simulink model "cpp_m1hp_demo"  (R2022b)
settings: Solver=FixedStepDiscrete  StartTime=0.0  StopTime=6  FixedStep=FEM_Ts  MaxStep=FEM_Ts  RelTol=1e-2
InitFcn:
  | %
  | % Initialization callback function
  | %
  | 
  | try
  |    fprintf('\nGMT IMS version (%s)!\n',simulink_fname );
  | 
  |    % Get Simulink model directory
  |    [filepath,name,ext] = fileparts(which(bdroot));
  | 
  |    if ~strcmp(filepath,pwd)
  |       fprintf('\nChanging current directory to \n %s \n',filepath);
  |       cd(filepath);
  |    end
  | 
  |    %
  |  if(osim.bpless_wl)
  |     fprintf('Generating bumpless wind load time series\n');
  |  end
  | catch
  |    warning('Running the InitFcn from puSimulate script');
  | end
values from neighbouring files (symbols this model uses):
  a_max = 250e-6    (= 0.00025)    [load_im_with_m1act_damp.m]    (also in load_m1hp_cpp_demo.m)
  b = B(:,in)*m1sys{seg}.Kbal    [evalM1ofl_act_damp.m]
  c = [Upsilon*C(out0,:);     C(out1a,:)-C(out1b,:);     C(out2,:)]    [evalM1ofl_act_damp.m]
  delta_sim = 1e-3    (= 0.001)    [load_im_with_m1act_damp.m]    (also in load_m1hp_cpp_demo.m)
  drv_delay = ceil(mount.delay/FEM_Ts)    [load_im_with_m1act_damp.m]    (also in load_m1hp_cpp_demo.m)
  FEM_Ts = 1/1e3    (= 0.001)    [load_im_with_m1act_damp.m]    (also in load_m1hp_cpp_demo.m)
  Hdrive_d = c2d(o.Hdrive(1,1), FEM_Ts, 'tustin')    [load_im_with_m1act_damp.m]    (also in load_m1hp_cpp_demo.m)
  m1sys = ovr_ofl_crtl(m1sys,seg)    [evalM1ofl_act_damp.m]    (also in load_im_with_m1act_damp.m = ovr_ofl_crtl(m1sys))
  o = fun_confBase(oTest)    [load_im_with_m1act_damp.m]    (also in load_m1hp_cpp_demo.m)
  PG = zeros(length(om2),6)    [load_im_with_m1act_damp.m]    (also in load_m1hp_cpp_demo.m)
  phiB = inputs2ModalF(mode_ind_vec,indDesInputs)    [load_im_with_m1act_damp.m]    (also in load_m1hp_cpp_demo.m)
  phiC = modalDisp2Outputs(indDesOutputs,mode_ind_vec)    [load_im_with_m1act_damp.m]    (also in load_m1hp_cpp_demo.m)
  Psi_ss = gainMatrix(indDesOutputs,indDesInputs) - K_ss    [load_im_with_m1act_damp.m]    (also in load_m1hp_cpp_demo.m)
  t_gd = 0*0.5    (= 0)    [load_im_with_m1act_damp.m]    (also in load_m1hp_cpp_demo.m)
  t_gd_v = 0*t_gd    (= 0)    [load_im_with_m1act_damp.m]    (also in load_m1hp_cpp_demo.m)
  Tcmd = 12    [load_im_with_m1act_damp.m]    (also in load_m1hp_cpp_demo.m)
  v0 = 0    [load_im_with_m1act_damp.m]    (also in load_m1hp_cpp_demo.m)
  v_max = 50e-6    (= 5e-05)    [load_im_with_m1act_damp.m]    (also in load_m1hp_cpp_demo.m)
  x0 = 0    [load_im_with_m1act_damp.m]    (also in load_m1hp_cpp_demo.m)
  x0_f = xf(end,:)    [load_im_with_m1act_damp.m]    (also in load_m1hp_cpp_demo.m)
undefined symbols (not defined in the file or in its folder): a, A_f, az, az_ff_en, B_f, C_f, D_f, DiscIntNeverNeededParam, el, gir, magnitude, mount, osim
libraries: simulink x8, ims_block_library x7, simulink_extras x2
(part 2 of 3)

== system cpp_m1hp_demo/M1 CPP/cmd_pre_proc/CPP with multi-axis coordination1 ==
  k : Inport
  k_acd : Inport  Port=2
  Demux1 : Demux  Outputs=3
  Dk_merge : Merge  Inputs=4  InitialOutput=0
  If Action Subsystem : Subsystem  TreatAsAtomicUnit=on
  If Action Subsystem1 : Subsystem  TreatAsAtomicUnit=on
  If Action Subsystem6 : Subsystem  TreatAsAtomicUnit=on
  If Action Subsystem__1 : Subsystem  TreatAsAtomicUnit=on
  If2 : If  NumInputs=2  IfExpression=(u1 == 0) | (u1 <= u2(1))  ElseIfExpressions=((u1 > u2(1)) & (u1 <= u2(2))), ((u1 > u2(2)) & (u1 <= u2(3))), (u1 > u2(3))  ShowElse=off
  Dk : Outport
  wires:
  k_acd/1 -> If2/2, Demux1/1
  k/1 -> If2/1
  Demux1/3 -> If Action Subsystem6/1(t_acd)
  If Action Subsystem__1/1(Dk) -> Dk_merge/3
  Demux1/1 -> If Action Subsystem1/1(t_a)
  If2/1 -> If Action Subsystem/Action
  If Action Subsystem/1(Dk) -> Dk_merge/1
  Demux1/2 -> If Action Subsystem__1/1(t_ac)
  If Action Subsystem1/1(Dk) -> Dk_merge/2
  If Action Subsystem6/1(Dk) -> Dk_merge/4
  Dk_merge/1 -> Dk/1
  If2/2 -> If Action Subsystem1/Action
  If2/3 -> If Action Subsystem__1/Action
  If2/4 -> If Action Subsystem6/Action

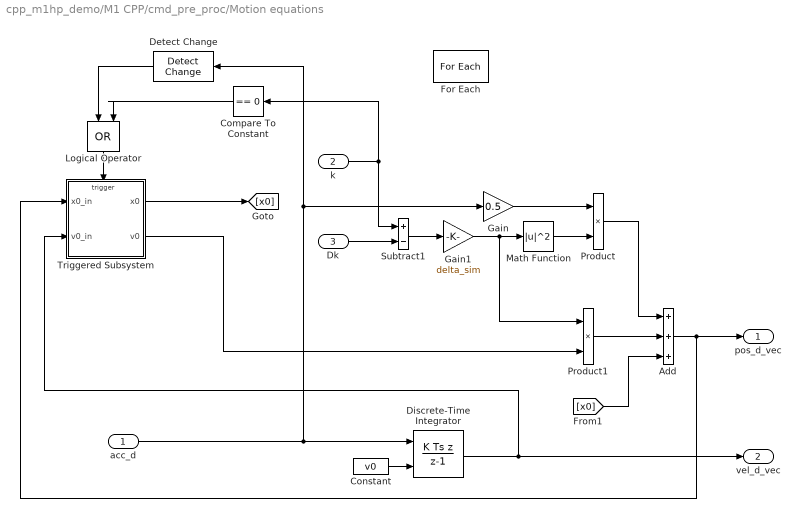
== system cpp_m1hp_demo/M1 CPP/cmd_pre_proc/Motion equations ==
  acc_d : Inport  Partition=on  PartitionDimension=1  PartitionWidth=1  PartitionOffset=0
  k : Inport  Port=2
  Dk : Inport  Port=3
  Add : Sum  Inputs=+++
  Compare To Constant : simulink/Logic and Bit Operations/Compare To Constant  relop===  const=0  OutDataTypeStr=boolean
  Constant : Constant  Value=v0
  Detect Change : simulink/Logic and Bit Operations/Detect Change  vinit=0  OutDataTypeStr=boolean
  Discrete-Time Integrator : DiscreteIntegrator  IntegratorMethod=Integration: Backward Euler  InitialConditionSource=external  InitialCondition=v0  SampleTime=-1  ICPrevOutput=DiscIntNeverNeededParam  ICPrevScaledInput=DiscIntNeverNeededParam
  For Each : ForEach  DisableCoverage=on
  Gain : Gain  Gain=0.5
  Gain1 : Gain  Gain=delta_sim  OutDataTypeStr=double
  Logical Operator : Logic  Operator=OR  IconShape=distinctive  AllPortsSameDT=off  OutDataTypeStr=boolean
  Math Function : Math  Operator=magnitude^2
  Product : Product
  Product1 : Product
  Subtract1 : Sum  Inputs=+-
  Triggered Subsystem : Subsystem  TreatAsAtomicUnit=on
  pos_d_vec : Outport  ConcatenationDimension=1
  vel_d_vec : Outport  Port=2  ConcatenationDimension=1
  wires:
  Detect Change/1 -> Logical Operator/1
  Add/1 -> pos_d_vec/1, Triggered Subsystem/1(x0_in)
  [x0] -> Add/3
  Gain/1 -> Product/1
  Constant/1 -> Discrete-Time Integrator/2
  Math Function/1 -> Product/2
  Triggered Subsystem/2(v0) -> Product1/2
  Product/1 -> Add/1
  acc_d/1 -> Discrete-Time Integrator/1, Gain/1, Detect Change/1
  Triggered Subsystem/1(x0) -> [x0]
  Discrete-Time Integrator/1 -> vel_d_vec/1, Triggered Subsystem/2(v0_in)
  Product1/1 -> Add/2
  k/1 -> Subtract1/1, Compare To Constant/1
  Gain1/1 -> Product1/1, Math Function/1
  Subtract1/1 -> Gain1/1
  Logical Operator/1 -> Triggered Subsystem/Trigger
  Compare To Constant/1 -> Logical Operator/2
  Dk/1 -> Subtract1/2

== system cpp_m1hp_demo/M1 CPP/cmd_pre_proc/Sample_generator ==
  Add : Sum
  Compare To Constant : simulink/Logic and Bit Operations/Compare To Constant  relop===  const=floor(Tcmd/delta_sim)  OutDataTypeStr=boolean
  Constant : Constant  OutDataTypeStr=uint32
  Resettable Delay : Delay  DelayLength=1  ExternalReset=Rising
      settings: InputPortMap=u0,r5
  Unit Delay : UnitDelay  SampleTime=-1  HasFrameUpgradeWarning=on
  k : Outport
  wires:
  Constant/1 -> Add/1
  Add/1 -> Resettable Delay/1, Unit Delay/1
  Resettable Delay/1 -> k/1, Add/2
  Compare To Constant/1 -> Resettable Delay/2
  Unit Delay/1 -> Compare To Constant/1

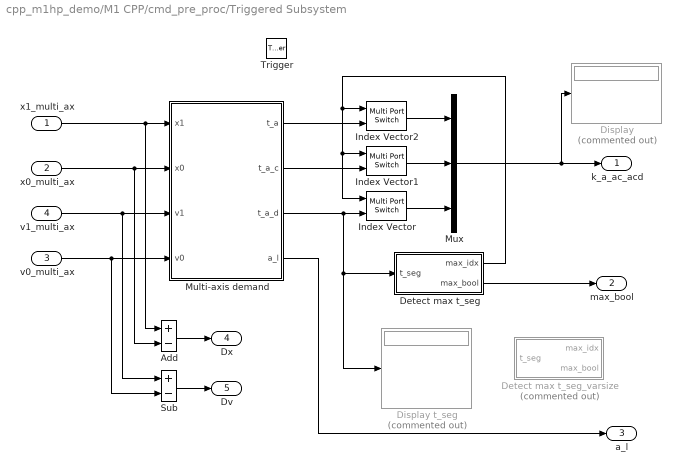
== system cpp_m1hp_demo/M1 CPP/cmd_pre_proc/Triggered Subsystem ==
  x1_multi_ax : Inport
  x0_multi_ax : Inport  Port=2  LatchByDelayingOutsideSignal=on
  v0_multi_ax : Inport  Port=3  LatchByDelayingOutsideSignal=on
  v1_multi_ax : Inport  Port=4
  Trigger : TriggerPort  VariantControl=Variant  InitialTriggerSignalState=zero
  Add : Sum  Inputs=+-
  Detect max t_seg : Subsystem
  Detect max t_seg_varsize : Subsystem  Commented=on
  Display : Display  Commented=on
  Display t_seg : Display  Commented=on
  Index Vector : MultiPortSwitch  Inputs=1  RndMeth=Simplest  SaturateOnIntegerOverflow=off
  Index Vector1 : MultiPortSwitch  Inputs=1  RndMeth=Simplest  SaturateOnIntegerOverflow=off
  Index Vector2 : MultiPortSwitch  Inputs=1  RndMeth=Simplest  SaturateOnIntegerOverflow=off
  Multi-axis demand : Subsystem  TreatAsAtomicUnit=on
  Mux : Mux  Inputs=3
  Sub : Sum  Inputs=+-
  k_a_ac_acd : Outport
  max_bool : Outport  Port=2
  a_l : Outport  Port=3
  Dx : Outport  Port=4
  Dv : Outport  Port=5
  wires:
  x1_multi_ax/1 -> Add/1, Multi-axis demand/1(x1)
  x0_multi_ax/1 -> Add/2, Multi-axis demand/2(x0)
  Detect max t_seg/1(max_idx) -> Index Vector1/1, Index Vector/1, Index Vector2/1
  v0_multi_ax/1 -> Sub/2, Multi-axis demand/4(v0)
  v1_multi_ax/1 -> Sub/1, Multi-axis demand/3(v1)
  Multi-axis demand/3(t_a_d) -> Index Vector/2, Display t_seg/1, Detect max t_seg/1(t_seg)
  Multi-axis demand/4(a_l) -> a_l/1
  Multi-axis demand/1(t_a) -> Index Vector2/2
  Multi-axis demand/2(t_a_c) -> Index Vector1/2
  Index Vector2/1 -> Mux/1
  Index Vector1/1 -> Mux/2
  Index Vector/1 -> Mux/3
  Mux/1 -> k_a_ac_acd/1, Display/1
  Add/1 -> Dx/1
  Sub/1 -> Dv/1
  Detect max t_seg/2(max_bool) -> max_bool/1

== system cpp_m1hp_demo/Mount_Drv_FDR2023_linear/DRV Friction/AZ DT Lugre Fr mode ==
  v : Inport
  Enable : EnablePort
  Constant : Constant  Value=iIsSig01Active
  Discrete-Time Integrator : DiscreteIntegrator  SampleTime=-1  ICPrevOutput=DiscIntNeverNeededParam  ICPrevScaledInput=DiscIntNeverNeededParam
  Sum : Sum  Inputs=+++
  g(v) : Subsystem
  sigma_0 : Gain  Gain=sigma0
  sigma_1 : Gain  Gain=sigma1
  sigma_v : Gain  Gain=sigmav
  v2z : Subsystem
  Tfr : Outport
  wires:
  Constant/1 -> g(v)/Enable, v2z/Enable
  v/1 -> sigma_v/1, v2z/1(v), g(v)/1(v)
  sigma_v/1 -> Sum/3
  sigma_1/1 -> Sum/1
  Sum/1 -> Tfr/1
  sigma_0/1 -> Sum/2
  g(v)/1(g) -> v2z/2(g(v))
  Discrete-Time Integrator/1 -> v2z/3(z), sigma_0/1
  v2z/1(dz) -> sigma_1/1, Discrete-Time Integrator/1

== system cpp_m1hp_demo/Mount_Drv_FDR2023_linear/DRV Friction/EL DT Lugre Fr model ==
  v : Inport
  Enable : EnablePort
  Constant : Constant  Value=iIsSig01Active
  Discrete-Time Integrator : DiscreteIntegrator  SampleTime=-1  ICPrevOutput=DiscIntNeverNeededParam  ICPrevScaledInput=DiscIntNeverNeededParam
  Sum : Sum  Inputs=+++
  g(v) : Subsystem
  sigma_0 : Gain  Gain=sigma0
  sigma_1 : Gain  Gain=sigma1
  sigma_v : Gain  Gain=sigmav
  v2z : Subsystem
  Tfr : Outport
  wires:
  Constant/1 -> g(v)/Enable, v2z/Enable
  sigma_0/1 -> Sum/2
  Discrete-Time Integrator/1 -> v2z/3(z), sigma_0/1
  g(v)/1(g) -> v2z/2(g(v))
  v/1 -> sigma_v/1, v2z/1(v), g(v)/1(v)
  Sum/1 -> Tfr/1
  sigma_1/1 -> Sum/1
  v2z/1(dz) -> sigma_1/1, Discrete-Time Integrator/1
  sigma_v/1 -> Sum/3

== system cpp_m1hp_demo/Mount_Drv_FDR2023_linear/DRV Friction/EL DT Lugre Fr model_ ==
  vel : Inport
  Enable : EnablePort
  Constant : Constant  Value=frParStruct.iIsSig01Active
  Discrete-Time Integrator : DiscreteIntegrator  SampleTime=-1  ICPrevOutput=DiscIntNeverNeededParam  ICPrevScaledInput=DiscIntNeverNeededParam
  Sum : Sum  Inputs=+++
  To Workspace : ToWorkspace  VariableName=el_Ve  SampleTime=-1
  To Workspace1 : ToWorkspace  VariableName=el_To  SampleTime=-1
  g(v) : Subsystem
  sigma_0 : Gain  Gain=frParStruct.sigm0
  sigma_1 : Gain  Gain=frParStruct.sigm1
  sigma_v : Gain  Gain=frParStruct.sigmv
  v2z : Subsystem
  FrTorque : Outport  VectorParamsAs1DForOutWhenUnconnected=off
  wires:
  Sum/1 -> FrTorque/1, To Workspace1/1
  v2z/1(dz) -> sigma_1/1, Discrete-Time Integrator/1
  Discrete-Time Integrator/1 -> v2z/3(z), sigma_0/1
  sigma_1/1 -> Sum/1
  g(v)/1(g) -> v2z/2(g(v))
  sigma_0/1 -> Sum/2
  Constant/1 -> v2z/Enable, g(v)/Enable
  vel/1 -> sigma_v/1, To Workspace/1, g(v)/1(v), v2z/1(v)
  sigma_v/1 -> Sum/3  "Viscose Friction"

== system cpp_m1hp_demo/Mount_Drv_FDR2023_linear/DRV Friction/GIR DT Lugre Fr model ==
  note: Discretized blocks
  v : Inport
  Enable : EnablePort
  Discrete Transfer Fcn : DiscreteTransferFcn  Numerator=[1 1]  Denominator="[1+(1/pi/20/FEM_Ts),  (1-(1/pi/20/FEM_Ts))]"  SampleTime=FEM_Ts
  Discrete-Time Integrator : DiscreteIntegrator  SampleTime=FEM_Ts  ICPrevOutput=DiscIntNeverNeededParam  ICPrevScaledInput=DiscIntNeverNeededParam
  Sum : Sum  Inputs=+++
  g(v) : Subsystem
  iIsSig01Active : Gain  Gain=iIsSig01Active
  on/off : Gain
  sigma_0 : Gain  Gain=sigma0
  sigma_1 : Gain  Gain=sigma1
  sigma_v : Gain  Gain=sigmav
  v2z : Subsystem
      settings: MinAlgLoopOccurrences=on
  Tfr : Outport
  wires:
  Discrete Transfer Fcn/1 -> sigma_1/1
  on/off/1 -> Sum/1
  sigma_1/1 -> on/off/1
  Sum/1 -> Tfr/1
  v/1 -> sigma_v/1, iIsSig01Active/1
  iIsSig01Active/1 -> v2z/1(v), g(v)/1(v)
  sigma_v/1 -> Sum/3
  sigma_0/1 -> Sum/2
  Discrete-Time Integrator/1 -> v2z/3(z), sigma_0/1
  v2z/1(dz) -> Discrete Transfer Fcn/1, Discrete-Time Integrator/1
  g(v)/1(g) -> v2z/2(g(v))

== system cpp_m1hp_demo/Mount_Drv_FDR2023_linear/DRV Friction/GIR DT Lugre Fr model_ ==
  vel : Inport
  Enable : EnablePort
  Discrete-Time Integrator : DiscreteIntegrator  SampleTime=-1  ICPrevOutput=DiscIntNeverNeededParam  ICPrevScaledInput=DiscIntNeverNeededParam
  Gain : Gain  Gain=frParStruct.iIsSig01Active
  Scope : Scope  Commented=on  NumInputPorts=2
  Scope1 : Scope  NumInputPorts=3
  Sum : Sum  Inputs=+++
  To Workspace : ToWorkspace  VariableName=gir_Ve  SampleTime=-1
  To Workspace1 : ToWorkspace  VariableName=gir_To  SampleTime=-1
  g(v) : Subsystem
  sigma_0 : Gain  Gain=frParStruct.sigm0
  sigma_1 : Gain  Gain=frParStruct.sigm1
  sigma_v : Gain  Gain=frParStruct.sigmv
  v2z : Subsystem
  FrTorque : Outport  VectorParamsAs1DForOutWhenUnconnected=off
  wires:
  sigma_1/1 -> Sum/1, Scope1/1  "sigma1*dz"
  sigma_0/1 -> Sum/2, Scope1/2  "sigma0*z"
  Gain/1 -> g(v)/1(v), v2z/1(v)
  Sum/1 -> FrTorque/1, To Workspace1/1
  v2z/1(dz) -> Scope/1, sigma_1/1, Discrete-Time Integrator/1  "dz"
  Discrete-Time Integrator/1 -> v2z/3(z), sigma_0/1, Scope/2  "z"
  g(v)/1(g) -> v2z/2(g(v))
  vel/1 -> sigma_v/1, To Workspace/1, Gain/1
  sigma_v/1 -> Sum/3, Scope1/3  "Viscous Friction"

== system cpp_m1hp_demo/Mount_Drv_FDR2023_linear/Friction/Friction Alt ==
  v : Inport
  Enable : EnablePort
  Constant : Constant  Value=iIsSig01Active
  Integrator2 : Integrator
  Sum : Sum  Inputs=+++
  g(v) : Subsystem
  sigma_0 : Gain  Gain=sigma0
  sigma_1 : Gain  Gain=sigma1
  sigma_v : Gain  Gain=sigmav
  v2z : Subsystem
  Tfr : Outport
  wires:
  v2z/1(dz) -> Integrator2/1, sigma_1/1
  Integrator2/1 -> sigma_0/1, v2z/3(z)
  g(v)/1(g) -> v2z/2(g(v))
  sigma_0/1 -> Sum/2
  Sum/1 -> Tfr/1
  sigma_1/1 -> Sum/1
  sigma_v/1 -> Sum/3
  v/1 -> g(v)/1(v), v2z/1(v), sigma_v/1
  Constant/1 -> v2z/Enable, g(v)/Enable

== system cpp_m1hp_demo/Mount_Drv_FDR2023_linear/Friction/Friction Az ==
  v : Inport
  Enable : EnablePort
  Constant : Constant  Value=iIsSig01Active
  Integrator2 : Integrator
  Sum : Sum  Inputs=+++
  g(v) : Subsystem
  sigma_0 : Gain  Gain=sigma0
  sigma_1 : Gain  Gain=sigma1
  sigma_v : Gain  Gain=sigmav
  v2z : Subsystem
  Tfr : Outport
  wires:
  v2z/1(dz) -> Integrator2/1, sigma_1/1
  Integrator2/1 -> sigma_0/1, v2z/3(z)
  g(v)/1(g) -> v2z/2(g(v))
  sigma_0/1 -> Sum/2
  Sum/1 -> Tfr/1
  sigma_1/1 -> Sum/1
  sigma_v/1 -> Sum/3
  v/1 -> g(v)/1(v), v2z/1(v), sigma_v/1
  Constant/1 -> g(v)/Enable, v2z/Enable

== system cpp_m1hp_demo/Mount_Drv_FDR2023_linear/Friction/Friction Gir ==
  v : Inport
  Enable : EnablePort
  Integrator2 : Integrator
  PT1 : Subsystem  mask{f=20}
      mask prompts: f "f(Hz)"
      mask Display: fprintf('PT1')
  Sum : Sum  Inputs=+++
  g(v) : Subsystem
  iIsSig01Active : Gain  Gain=iIsSig01Active
  on/off : Gain
  sigma_0 : Gain  Gain=sigma0
  sigma_1 : Gain  Gain=sigma1
  sigma_v : Gain  Gain=sigmav
  v2z : Subsystem
      settings: MinAlgLoopOccurrences=on
  Tfr : Outport
  wires:
  g(v)/1(g) -> v2z/2(g(v))
  v2z/1(dz) -> PT1/1(in), Integrator2/1
  Integrator2/1 -> sigma_0/1, v2z/3(z)
  sigma_0/1 -> Sum/2
  sigma_v/1 -> Sum/3
  iIsSig01Active/1 -> g(v)/1(v), v2z/1(v)
  v/1 -> iIsSig01Active/1, sigma_v/1
  Sum/1 -> Tfr/1
  sigma_1/1 -> on/off/1
  on/off/1 -> Sum/1
  PT1/1(out) -> sigma_1/1

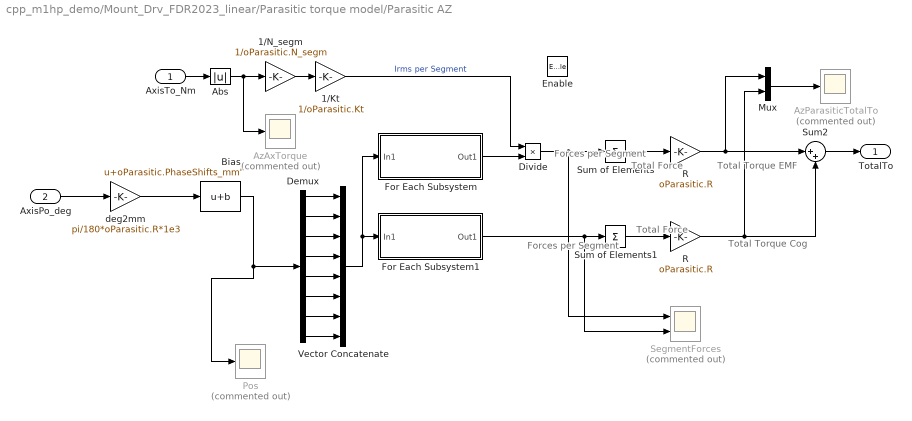
== system cpp_m1hp_demo/Mount_Drv_FDR2023_linear/Parasitic torque model/Parasitic AZ ==
  note: Total
      | Torque Cog
  note: Total
      | Torque EMF
  note: Total
      | Force
  note: Forces per
      | Segment
  note: Forces per
      | Segment
  note: Total
      | Force
  AxisTo_Nm : Inport
  AxisPo_deg : Inport  Port=2
  Enable : EnablePort
  1/Kt : Gain  Gain=1/oParasitic.Kt
  1/N_segm : Gain  Gain=1/oParasitic.N_segm
  Abs : Abs  SaturateOnIntegerOverflow=off
  AzAxTorque : Scope  Commented=on
  AzParasiticTotalTo : Scope  Commented=on
  Bias : Bias  Bias=oParasitic.PhaseShifts_mm'  SaturateOnIntegerOverflow=off
  Demux : Demux  Outputs=8
  Divide : Product  Inputs=**
  For Each Subsystem : Subsystem  TreatAsAtomicUnit=on
  For Each Subsystem1 : Subsystem  TreatAsAtomicUnit=on
  Mux : Mux  Inputs=2
  Pos : Scope  Commented=on
  R : Gain  Gain=oParasitic.R
  "R " : Gain  Gain=oParasitic.R
  SegmentForces : Scope  Commented=on  NumInputPorts=2
  Sum of Elements : Sum  Inputs=+
  Sum of Elements1 : Sum  Inputs=+
  Sum2 : Sum  Inputs=|++
  Vector Concatenate : Concatenate  NumInputs=oParasitic.N_segm
  deg2mm : Gain  Gain=pi/180*oParasitic.R*1e3
  TotalTo : Outport
  wires:
  AxisPo_deg/1 -> deg2mm/1
  deg2mm/1 -> Bias/1
  Abs/1 -> 1/N_segm/1, AzAxTorque/1
  AxisTo_Nm/1 -> Abs/1
  Demux/8 -> Vector Concatenate/8
  Demux/7 -> Vector Concatenate/7
  Demux/6 -> Vector Concatenate/6
  Demux/5 -> Vector Concatenate/5
  Demux/4 -> Vector Concatenate/4
  Demux/3 -> Vector Concatenate/3
  Demux/2 -> Vector Concatenate/2
  Demux/1 -> Vector Concatenate/1
  For Each Subsystem1/1(Out1) -> Sum of Elements1/1, SegmentForces/2
  For Each Subsystem/1(Out1) -> Divide/2
  Vector Concatenate/1 -> For Each Subsystem1/1(In1), For Each Subsystem/1(In1)
  Bias/1 -> Pos/1, Demux/1
  Mux/1 -> AzParasiticTotalTo/1
  1/Kt/1 -> Divide/1  "Irms per Segment"
  Sum of Elements/1 -> R/1
  1/N_segm/1 -> 1/Kt/1
  R/1 -> Sum2/1, Mux/1
  "R "/1 -> Mux/2, Sum2/2
  Divide/1 -> SegmentForces/1, Sum of Elements/1
  Sum2/1 -> TotalTo/1
  Sum of Elements1/1 -> "R "/1

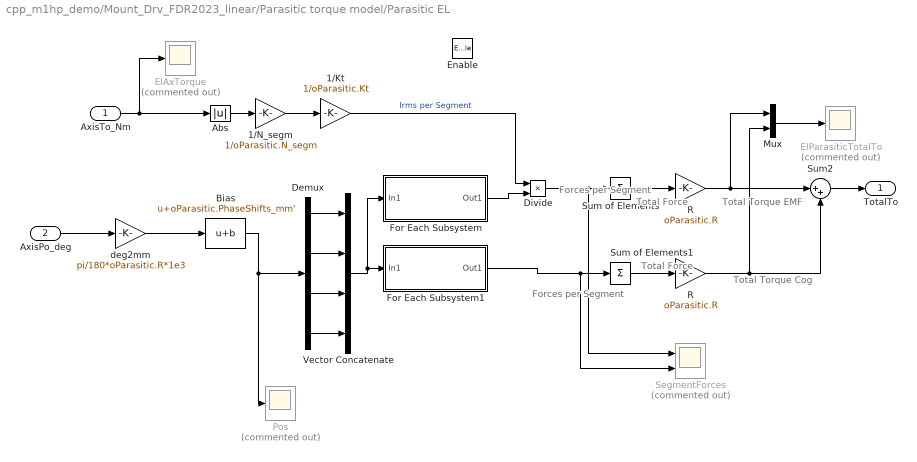
== system cpp_m1hp_demo/Mount_Drv_FDR2023_linear/Parasitic torque model/Parasitic EL ==
  note: Total
      | Torque Cog
  note: Total
      | Torque EMF
  note: Total
      | Force
  note: Forces per
      | Segment
  note: Forces per
      | Segment
  note: Total
      | Force
  AxisTo_Nm : Inport
  AxisPo_deg : Inport  Port=2
  Enable : EnablePort
  1/Kt : Gain  Gain=1/oParasitic.Kt
  1/N_segm : Gain  Gain=1/oParasitic.N_segm
  Abs : Abs  SaturateOnIntegerOverflow=off
  Bias : Bias  Bias=oParasitic.PhaseShifts_mm'  SaturateOnIntegerOverflow=off
  Demux : Demux  Outputs=oParasitic.N_segm
  Divide : Product  Inputs=**
  ElAxTorque : Scope  Commented=on
  ElParasiticTotalTo : Scope  Commented=on
  For Each Subsystem : Subsystem  TreatAsAtomicUnit=on
  For Each Subsystem1 : Subsystem  TreatAsAtomicUnit=on
  Mux : Mux  Inputs=2
  Pos : Scope  Commented=on
  R : Gain  Gain=oParasitic.R
  "R " : Gain  Gain=oParasitic.R
  SegmentForces : Scope  Commented=on  NumInputPorts=2
  Sum of Elements : Sum  Inputs=+
  Sum of Elements1 : Sum  Inputs=+
  Sum2 : Sum  Inputs=|++
  Vector Concatenate : Concatenate  NumInputs=oParasitic.N_segm
  deg2mm : Gain  Gain=pi/180*oParasitic.R*1e3
  TotalTo : Outport
  wires:
  AxisPo_deg/1 -> deg2mm/1
  deg2mm/1 -> Bias/1
  Abs/1 -> 1/N_segm/1
  AxisTo_Nm/1 -> Abs/1, ElAxTorque/1
  Demux/4 -> Vector Concatenate/4
  Demux/3 -> Vector Concatenate/3
  Demux/2 -> Vector Concatenate/2
  Demux/1 -> Vector Concatenate/1
  For Each Subsystem1/1(Out1) -> Sum of Elements1/1, SegmentForces/2
  For Each Subsystem/1(Out1) -> Divide/2
  Vector Concatenate/1 -> For Each Subsystem1/1(In1), For Each Subsystem/1(In1)
  Bias/1 -> Demux/1, Pos/1
  Mux/1 -> ElParasiticTotalTo/1
  1/Kt/1 -> Divide/1  "Irms per Segment"
  Sum of Elements/1 -> R/1
  1/N_segm/1 -> 1/Kt/1
  R/1 -> Sum2/1, Mux/1
  "R "/1 -> Mux/2, Sum2/2
  Divide/1 -> SegmentForces/1, Sum of Elements/1
  Sum2/1 -> TotalTo/1
  Sum of Elements1/1 -> "R "/1

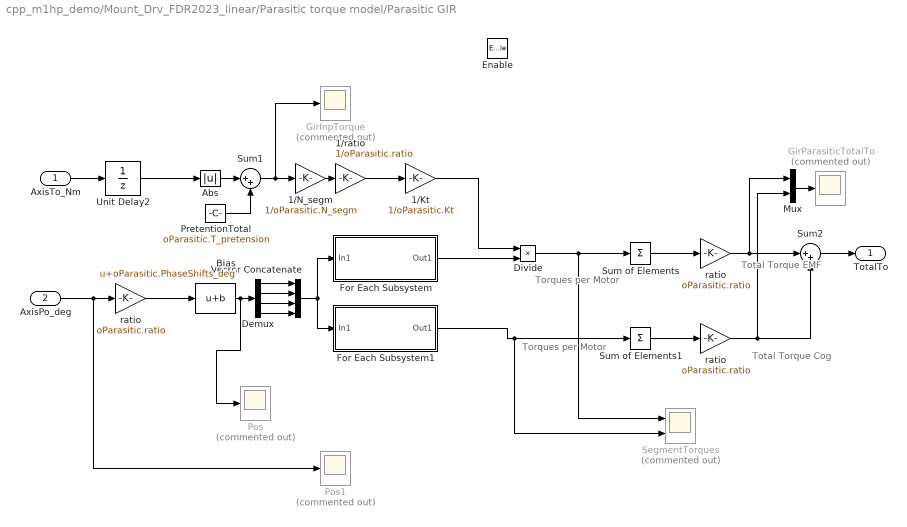
== system cpp_m1hp_demo/Mount_Drv_FDR2023_linear/Parasitic torque model/Parasitic GIR ==
  note: Total
      | Torque Cog
  note: Total
      | Torque EMF
  note: Torques
      | per Motor
  note: Torques per
      | Motor
  AxisTo_Nm : Inport
  AxisPo_deg : Inport  Port=2
  Enable : EnablePort
  1/Kt : Gain  Gain=1/oParasitic.Kt
  1/N_segm : Gain  Gain=1/oParasitic.N_segm
  "1/ratio   " : Gain  Gain=1/oParasitic.ratio
  Abs : Abs  SaturateOnIntegerOverflow=off
  Bias : Bias  Bias=oParasitic.PhaseShifts_deg'  SaturateOnIntegerOverflow=off
  Demux : Demux
  Divide : Product  Inputs=**
  For Each Subsystem : Subsystem  TreatAsAtomicUnit=on
  For Each Subsystem1 : Subsystem  TreatAsAtomicUnit=on
  GirInpTorque : Scope  Commented=on
  GirParasiticTotalTo : Scope  Commented=on
  Mux : Mux  Inputs=2
  Pos : Scope  Commented=on
  Pos1 : Scope  Commented=on
  PretentionTotal : Constant  Value=oParasitic.T_pretension
  SegmentTorques : Scope  Commented=on  NumInputPorts=2
  Sum of Elements : Sum  Inputs=+
  Sum of Elements1 : Sum  Inputs=+
  Sum1 : Sum  Inputs=|++
  Sum2 : Sum  Inputs=|++
  Unit Delay2 : UnitDelay  SampleTime=-1  HasFrameUpgradeWarning=on
  Vector Concatenate : Concatenate  NumInputs=oParasitic.N_segm
  ratio : Gain  Gain=oParasitic.ratio
  "ratio " : Gain  Gain=oParasitic.ratio
  "ratio  " : Gain  Gain=oParasitic.ratio
  TotalTo : Outport
  wires:
  Unit Delay2/1 -> Abs/1
  AxisTo_Nm/1 -> Unit Delay2/1
  Sum1/1 -> 1/N_segm/1, GirInpTorque/1
  1/Kt/1 -> Divide/1
  PretentionTotal/1 -> Sum1/2
  Abs/1 -> Sum1/1
  "1/ratio   "/1 -> 1/Kt/1
  1/N_segm/1 -> "1/ratio   "/1
  Bias/1 -> Demux/1, Pos/1
  Demux/4 -> Vector Concatenate/4
  Demux/3 -> Vector Concatenate/3
  Demux/2 -> Vector Concatenate/2
  Demux/1 -> Vector Concatenate/1
  Vector Concatenate/1 -> For Each Subsystem1/1(In1), For Each Subsystem/1(In1)
  For Each Subsystem/1(Out1) -> Divide/2
  For Each Subsystem1/1(Out1) -> Sum of Elements1/1, SegmentTorques/2
  "ratio  "/1 -> Sum2/1, Mux/1
  "ratio "/1 -> Mux/2, Sum2/2
  Sum of Elements/1 -> "ratio  "/1
  Sum of Elements1/1 -> "ratio "/1
  ratio/1 -> Bias/1
  AxisPo_deg/1 -> ratio/1, Pos1/1
  Mux/1 -> GirParasiticTotalTo/1
  Divide/1 -> Sum of Elements/1, SegmentTorques/1
  Sum2/1 -> TotalTo/1

== system cpp_m1hp_demo/Mount_Drv_FDR2023_linear/ToothContact Torques/ToothContact GIR (Norm) ==
  AxisPos_deg : Inport
  AxisTo : Inport  Port=2
  1-D Lookup Table : Lookup_n-D  NumberOfTableDimensions=1  BreakpointsForDimension1=oToothContact.oInterp.Pos  Table=oToothContact.oInterp.TorqueRate  InternalRulePriority=Speed  RndMeth=Simplest
  Abs : Abs  SaturateOnIntegerOverflow=off
  Gain : Gain  Gain=0.25
  Max Position : Constant  Value=oToothContact.maxPos
  Phase Shifts : Constant  Value=oToothContact.PhaseShift_deg
  PretensionTotal : Constant  Value=gir.T_pretension
  Product1 : Product  RndMeth=Zero
  Rem : Math  Operator=rem
  Sum of Elements : Sum  Inputs=+  CollapseMode=Specified dimension
  Sum1 : Sum  Inputs=|++
  Sum2 : Sum  Inputs=|++
  TotalTo : Outport
  wires:
  AxisTo/1 -> Abs/1
  Gain/1 -> Product1/2
  Sum1/1 -> Gain/1
  PretensionTotal/1 -> Sum1/2
  Abs/1 -> Sum1/1
  AxisPos_deg/1 -> Sum2/1
  Sum of Elements/1 -> TotalTo/1
  Phase Shifts/1 -> Sum2/2
  Sum2/1 -> Rem/1
  1-D Lookup Table/1 -> Product1/1
  Rem/1 -> 1-D Lookup Table/1
  Max Position/1 -> Rem/2
  Product1/1 -> Sum of Elements/1  "Position"

== system cpp_m1hp_demo/Mount_Drv_FDR2023_linear/ToothContact Torques/ToothContact GIR (Peak) ==
  AxisPos_deg : Inport
  AxisTo : Inport  Port=2
  1-D Lookup Table : Lookup_n-D  NumberOfTableDimensions=1  BreakpointsForDimension1=oToothContact.oInterp.Pos  Table=oToothContact.oInterp.TorqueRate  InternalRulePriority=Speed  RndMeth=Simplest
  Abs : Abs  SaturateOnIntegerOverflow=off
  Gain : Gain  Gain=0.25
  Max Position : Constant  Value=oToothContact.maxPos
  Phase Shifts : Constant  Value=oToothContact.PhaseShift_deg
  PretensionTotal : Constant  Value=gir.T_pretension
  Product1 : Product  RndMeth=Zero
  Rem : Math  Operator=rem
  Sum of Elements : Sum  Inputs=+  CollapseMode=Specified dimension
  Sum1 : Sum  Inputs=|++
  Sum2 : Sum  Inputs=|++
  TotalTo : Outport
  wires:
  AxisTo/1 -> Abs/1
  Gain/1 -> Product1/2
  Sum1/1 -> Gain/1
  PretensionTotal/1 -> Sum1/2
  Abs/1 -> Sum1/1
  AxisPos_deg/1 -> Sum2/1
  Sum of Elements/1 -> TotalTo/1
  Phase Shifts/1 -> Sum2/2
  Sum2/1 -> Rem/1
  1-D Lookup Table/1 -> Product1/1
  Rem/1 -> 1-D Lookup Table/1
  Max Position/1 -> Rem/2
  Product1/1 -> Sum of Elements/1  "Position"

== system cpp_m1hp_demo/Telescope model/Structural Dynamics GMT/FEM_SS ==
  note: 2nd order form simulation
  In : Inport
  Sum2 : Sum  Inputs=+++
  Sum3 : Sum  Inputs=+++
  Unit Delay : UnitDelay  SampleTime=FEM_Ts  HasFrameUpgradeWarning=on
  Unit Delay1 : UnitDelay  SampleTime=FEM_Ts  HasFrameUpgradeWarning=on
  gamma1 : Gain  Gain=PG(:,3)
  gamma2 : Gain  Gain=PG(:,6)
  phi11 : Gain  Gain=PG(:,1)
  phi12 : Gain  Gain=PG(:,2)
  phi21 : Gain  Gain=PG(:,4)
  phi22 : Gain  Gain=PG(:,5)
  phiB : Gain  Gain=phiB  Multiplication=Matrix(K*u) (u vector)
  phiC : Gain  Gain=phiC  Multiplication=Matrix(K*u) (u vector)
  pos : Outport  VectorParamsAs1DForOutWhenUnconnected=off
  wires:
  In/1 -> phiB/1
  phiC/1 -> pos/1
  phiB/1 -> gamma1/1, gamma2/1
  Unit Delay1/1 -> phi22/1, phi12/1
  phi11/1 -> Sum3/3
  gamma1/1 -> Sum3/1
  phi22/1 -> Sum2/1
  phi21/1 -> Sum2/2
  gamma2/1 -> Sum2/3
  Sum3/1 -> Unit Delay/1
  Sum2/1 -> Unit Delay1/1
  phi12/1 -> Sum3/2
  Unit Delay/1 -> phiC/1, phi21/1, phi11/1

== system cpp_m1hp_demo/M1 CPP/cmd_pre_proc/Bessel filter/Jerk-limitation ==
  acc : Inport
  vel : Inport  Port=2
  pos : Inport  Port=3
  Add1 : Sum  Inputs=+++
  Add2 : Sum
  Bessel filter Acc : DiscreteStateSpace  A=A_f  B=B_f  C=C_f  D=D_f  InitialCondition=x0_f * 0  SampleTime=delta_sim
  Bessel filter Pos : DiscreteStateSpace  A=A_f  B=B_f  C=C_f  D=D_f  InitialCondition=x0_f * x0  SampleTime=delta_sim
  Bessel filter Vel : DiscreteStateSpace  A=A_f  B=B_f  C=C_f  D=D_f  InitialCondition=x0_f * v0  SampleTime=delta_sim
  Gain1 : Gain  Gain=t_gd
  Gain2 : Gain  Gain=t_gd_v
  Gain3 : Gain  Gain=t_gd^2
  acc_f : Outport
  vel_f : Outport  Port=2
  pos_f : Outport  Port=3
  wires:
  pos/1 -> Add1/2
  Bessel filter Pos/1 -> pos_f/1
  Bessel filter Acc/1 -> acc_f/1
  vel/1 -> Add2/2, Gain1/1
  Add2/1 -> Bessel filter Vel/1
  acc/1 -> Gain3/1, Bessel filter Acc/1, Gain2/1
  Bessel filter Vel/1 -> vel_f/1
  Gain2/1 -> Add2/1
  Gain1/1 -> Add1/1
  Gain3/1 -> Add1/3
  Add1/1 -> Bessel filter Pos/1

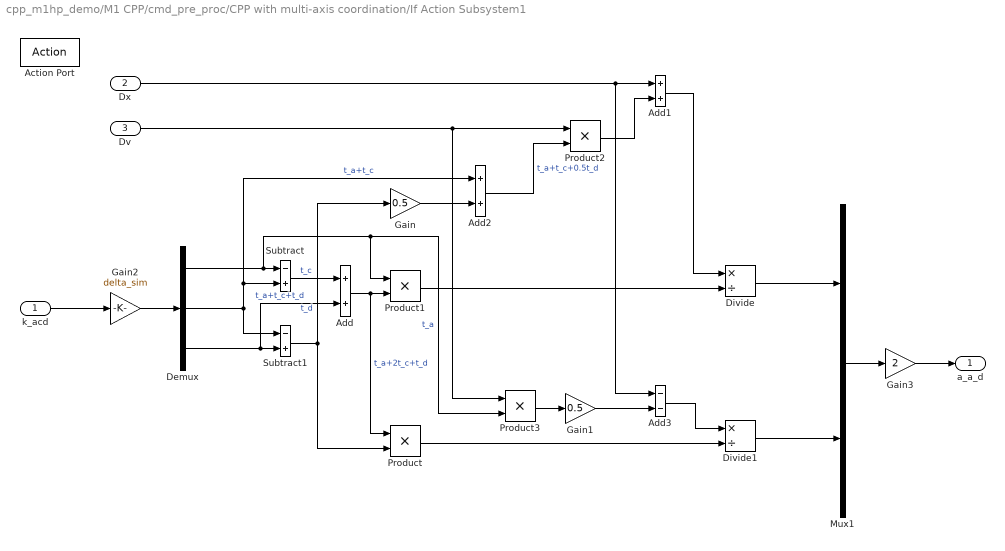
== system cpp_m1hp_demo/M1 CPP/cmd_pre_proc/CPP with multi-axis coordination/If Action Subsystem1 ==
  k_acd : Inport
  Dx : Inport  Port=2
  Dv : Inport  Port=3
  Action Port : ActionPort  ActionPortLabel=if(~u1 & (u2 == 1))
  Add : Sum
  Add1 : Sum
  Add2 : Sum
  Add3 : Sum  Inputs=--
  Demux : Demux  Outputs=3
  Divide : Product  Inputs=*/
  Divide1 : Product  Inputs=*/
  Gain : Gain  Gain=0.5
  Gain1 : Gain  Gain=0.5
  Gain2 : Gain  Gain=delta_sim  OutDataTypeStr=double
  Gain3 : Gain  Gain=2
  Mux1 : Mux  Inputs=2
  Product{,1..3} (4 alike) : Product
  Subtract : Sum  Inputs=-+
  Subtract1 : Sum  Inputs=-+
  a_a_d : Outport
  wires:
  Gain3/1 -> a_a_d/1
  Divide1/1 -> Mux1/2
  Demux/3 -> Add/2, Subtract1/2  "t_a+t_c+t_d"
  Add2/1 -> Product2/2  "t_a+t_c+0.5t_d"
  Gain1/1 -> Add3/2
  Product2/1 -> Add1/2
  Divide/1 -> Mux1/1
  Add3/1 -> Divide1/1
  Mux1/1 -> Gain3/1
  Product3/1 -> Gain1/1
  Product/1 -> Divide1/2
  Subtract/1 -> Add/1  "t_c"
  Dv/1 -> Product3/1, Product2/1
  Dx/1 -> Add3/1, Add1/1
  Add/1 -> Product/1, Product1/2  "t_a+2t_c+t_d"
  Demux/1 -> Product3/2, Product1/1, Subtract/1  "t_a"
  Product1/1 -> Divide/2
  Gain/1 -> Add2/2
  Subtract1/1 -> Gain/1, Product/2  "t_d"
  Demux/2 -> Subtract1/1, Add2/1, Subtract/2  "t_a+t_c"
  Add1/1 -> Divide/1
  k_acd/1 -> Gain2/1
  Gain2/1 -> Demux/1

== system cpp_m1hp_demo/M1 CPP/cmd_pre_proc/CPP with multi-axis coordination/If Action Subsystem2 ==
  acc_max_d : Inport
  Action Port : ActionPort  ActionPortLabel=else
  Mux : Mux  Inputs=2
  Unary Minus : UnaryMinus
  a_a_d : Outport
  wires:
  acc_max_d/1 -> Unary Minus/1, Mux/1
  Mux/1 -> a_a_d/1
  Unary Minus/1 -> Mux/2

== system cpp_m1hp_demo/M1 CPP/cmd_pre_proc/CPP with multi-axis coordination/If Action Subsystem3 ==
  Action Port : ActionPort  ActionPortLabel=elseif(~u1 & (u2 == 0))
  Constant : Constant  Value=0
  Mux : Mux  Inputs=2
  a_a_d : Outport
  wires:
  Mux/1 -> a_a_d/1
  Constant/1 -> Mux/2, Mux/1

== system cpp_m1hp_demo/M1 CPP/cmd_pre_proc/CPP with multi-axis coordination/If Action Subsystem4 ==
  Action Port : ActionPort  ActionPortLabel=if((u1 == 0))
  Constant : Constant  Value=0
  ac0 : Outport  VectorParamsAs1DForOutWhenUnconnected=off
  wires:
  Constant/1 -> ac0/1

== system cpp_m1hp_demo/M1 CPP/cmd_pre_proc/CPP with multi-axis coordination/If Action Subsystem5 ==
  Action Port : ActionPort  ActionPortLabel=elseif( ((u1 > u2(1)) & (u1 <= u2(2))))
  Constant : Constant  Value=0
  ac0 : Outport  VectorParamsAs1DForOutWhenUnconnected=off
  wires:
  Constant/1 -> ac0/1

== system cpp_m1hp_demo/M1 CPP/cmd_pre_proc/CPP with multi-axis coordination/If Action Subsystem6 ==
  Action Port : ActionPort  ActionPortLabel=elseif( (u1 > u2(3)))
  Constant : Constant  Value=0
  ac0 : Outport  VectorParamsAs1DForOutWhenUnconnected=off
  wires:
  Constant/1 -> ac0/1

== system cpp_m1hp_demo/M1 CPP/cmd_pre_proc/CPP with multi-axis coordination/If Action Subsystem_1 ==
  a_l : Inport
  Action Port : ActionPort  ActionPortLabel=elseif((u1 <= u2(1)))
  acc : Outport  InitialOutput=0  VectorParamsAs1DForOutWhenUnconnected=off
  wires:
  a_l/1 -> acc/1

== system cpp_m1hp_demo/M1 CPP/cmd_pre_proc/CPP with multi-axis coordination/If Action Subsystem__1 ==
  a_l : Inport
  Action Port : ActionPort  ActionPortLabel=elseif( ((u1 > u2(2)) & (u1 <= u2(3))))
  a_dec : Outport  InitialOutput=0  VectorParamsAs1DForOutWhenUnconnected=off
  wires:
  a_l/1 -> a_dec/1

== system cpp_m1hp_demo/M1 CPP/cmd_pre_proc/CPP with multi-axis coordination1/If Action Subsystem ==
  Action Port : ActionPort  ActionPortLabel=if((u1 == 0) | (u1 <= u2(1)))
  Constant1 : Constant  Value=0  OutDataTypeStr=uint32
  Dk : Outport  VectorParamsAs1DForOutWhenUnconnected=off
  wires:
  Constant1/1 -> Dk/1

== system cpp_m1hp_demo/M1 CPP/cmd_pre_proc/CPP with multi-axis coordination1/If Action Subsystem1 ==
  t_a : Inport
  Action Port : ActionPort  ActionPortLabel=elseif(((u1 > u2(1)) & (u1 <= u2(2))))
  Dk : Outport  InitialOutput=0  VectorParamsAs1DForOutWhenUnconnected=off
  wires:
  t_a/1 -> Dk/1

== system cpp_m1hp_demo/M1 CPP/cmd_pre_proc/CPP with multi-axis coordination1/If Action Subsystem6 ==
  t_acd : Inport
  Action Port : ActionPort  ActionPortLabel=elseif( (u1 > u2(3)))
  Dk : Outport  InitialOutput=0  VectorParamsAs1DForOutWhenUnconnected=off
  wires:
  t_acd/1 -> Dk/1

== system cpp_m1hp_demo/M1 CPP/cmd_pre_proc/CPP with multi-axis coordination1/If Action Subsystem__1 ==
  t_ac : Inport
  Action Port : ActionPort  ActionPortLabel=elseif( ((u1 > u2(2)) & (u1 <= u2(3))))
  Dk : Outport  InitialOutput=0  VectorParamsAs1DForOutWhenUnconnected=off
  wires:
  t_ac/1 -> Dk/1

== system cpp_m1hp_demo/M1 CPP/cmd_pre_proc/Motion equations/Triggered Subsystem ==
  x0_in : Inport  LatchByDelayingOutsideSignal=on
  v0_in : Inport  Port=2  LatchByDelayingOutsideSignal=on
  Trigger : TriggerPort  VariantControl=Variant
  x0 : Outport  SourceOfInitialOutputValue=Input signal  InitialOutput=[x0]  VectorParamsAs1DForOutWhenUnconnected=off
  v0 : Outport  Port=2  InitialOutput=[v0]  VectorParamsAs1DForOutWhenUnconnected=off
  wires:
  x0_in/1 -> x0/1
  v0_in/1 -> v0/1

== system cpp_m1hp_demo/M1 CPP/cmd_pre_proc/Triggered Subsystem/Detect max t_seg ==
  note: initially outputs idx 1
  t_seg : Inport
  Add : Sum  Inputs=+-
  Compare To Zero : simulink/Logic and Bit Operations/Compare To Zero  relop===  OutDataTypeStr=boolean
  For Iterator : ForIterator  ResetStates=reset  IterationSource=external  IterationLimit=3  IndexMode=Zero-based  IterationVariableDataType=int16
  Memory1 : Memory  InitialCondition=int16(1)  InheritSampleTime=on
  MinMax : MinMax  Function=max
  Selector1 : Selector  IndexOptions=Index vector (port)  Indices=[1 3]  OutputSizes=1
  Subtract : Sum  Inputs=+-  OutDataTypeStr=int32  RndMeth=Simplest
  Switch1 : Switch  Criteria=u2 ~= 0  SaturateOnIntegerOverflow=off  InputSameDT=off
  Width1 : Width  DataType=int16
  max_idx : Outport
  max_bool : Outport  Port=2
  wires:
  Width1/1 -> For Iterator/1, Add/1
  Switch1/1 -> Memory1/1, max_idx/1
  For Iterator/1 -> Add/2
  Add/1 -> Switch1/1, Selector1/2  "ii"
  Memory1/1 -> Switch1/3  "idxMinMax"
  Selector1/1 -> Switch1/2  "array(ii)"
  Subtract/1 -> Compare To Zero/1
  t_seg/1 -> Width1/1, MinMax/1, Subtract/1
  MinMax/1 -> Subtract/2
  Compare To Zero/1 -> Selector1/1, max_bool/1

== system cpp_m1hp_demo/M1 CPP/cmd_pre_proc/Triggered Subsystem/Detect max t_seg_varsize ==
  t_seg : Inport
  Compare To Zero : simulink/Logic and Bit Operations/Compare To Zero  relop===  OutDataTypeStr=boolean
  Display t_seg : Display  Commented=on
  Find Nonzero Elements : Find  NumberOfInputDimensions=3  OutDataTypeStr=uint8
  Index Vector : MultiPortSwitch  Commented=on  Inputs=1  SaturateOnIntegerOverflow=off  InputSameDT=off
  MinMax : MinMax  Function=max
  MinMax1 : MinMax
  Subtract : Sum  Inputs=+-  OutDataTypeStr=int32  RndMeth=Simplest
  max_idx : Outport
  max_bool : Outport  Port=2
  wires:
  MinMax/1 -> Subtract/2
  Subtract/1 -> Compare To Zero/1
  Find Nonzero Elements/1 -> MinMax1/1
  MinMax1/1 -> max_idx/1, Index Vector/1
  t_seg/1 -> Index Vector/2, Subtract/1, MinMax/1
  Compare To Zero/1 -> max_bool/1, Display t_seg/1, Find Nonzero Elements/1

== system cpp_m1hp_demo/M1 CPP/cmd_pre_proc/Triggered Subsystem/Multi-axis demand ==
  x1 : Inport  Partition=on  PartitionDimension=1  PartitionWidth=1  PartitionOffset=0
  x0 : Inport  Port=2  Partition=on  PartitionDimension=1  PartitionWidth=1  PartitionOffset=0
  v1 : Inport  Port=3  Partition=on  PartitionDimension=1  PartitionWidth=1  PartitionOffset=0
  v0 : Inport  Port=4  Partition=on  PartitionDimension=1  PartitionWidth=1  PartitionOffset=0
  Add : Sum
  Add_acd : Sum
  Constant : Constant  Value=a_max
  Constant1 : Constant  Value=v_max
  For Each : ForEach  DisableCoverage=on
  Gain1 : Gain  Gain=1/delta_sim  OutDataTypeStr=uint32
  Gain2 : Gain  Gain=1/delta_sim  OutDataTypeStr=uint32
  Gain3 : Gain  Gain=1/delta_sim  OutDataTypeStr=uint32
  MATLAB Function : MATLAB Function  TreatAsAtomicUnit=on
  t_a : Outport  ConcatenationDimension=1
  t_a_c : Outport  Port=2  ConcatenationDimension=1
  t_a_d : Outport  Port=3  ConcatenationDimension=1
  a_l : Outport  Port=4  ConcatenationDimension=1
  wires:
  x1/1 -> MATLAB Function/1(x1)
  Constant1/1 -> MATLAB Function/3(v_max)
  x0/1 -> MATLAB Function/5(x0)
  v0/1 -> MATLAB Function/6(v0)
  MATLAB Function/4(a_l) -> a_l/1
  Constant/1 -> MATLAB Function/4(a_max)
  v1/1 -> MATLAB Function/2(v1)
  Gain2/1 -> Add/2
  Add/1 -> t_a_c/1, Add_acd/1
  MATLAB Function/2(t_c) -> Gain2/1
  Gain3/1 -> Add_acd/2
  Add_acd/1 -> t_a_d/1
  MATLAB Function/1(t_a) -> Gain1/1
  MATLAB Function/3(t_d) -> Gain3/1
  Gain1/1 -> t_a/1, Add/1

== system cpp_m1hp_demo/Mount_Drv_FDR2023_linear/DRV Friction/AZ DT Lugre Fr mode/g(v) ==
  v : Inport
  Enable : EnablePort
  Constant : Constant  Value=0
  Sum : Sum  Inputs=|++
  gc : Constant  Value=Tc/sigma0
  gs : Subsystem
  g : Outport
  wires:
  Constant/1 -> gs/Enable
  gc/1 -> Sum/2
  gs/1(gs(v)) -> Sum/1
  v/1 -> gs/1(v)
  Sum/1 -> g/1

== system cpp_m1hp_demo/Mount_Drv_FDR2023_linear/DRV Friction/AZ DT Lugre Fr mode/v2z ==
  v : Inport
  g(v) : Inport  Port=2
  z : Inport  Port=3
  Enable : EnablePort
  Abs : Abs  SaturateOnIntegerOverflow=off
  Divide : Product  Inputs=*/*
  Sum : Sum  Inputs=|+-
  dz : Outport
  wires:
  z/1 -> Divide/3
  g(v)/1 -> Divide/2
  Sum/1 -> dz/1
  v/1 -> Abs/1, Sum/1
  Divide/1 -> Sum/2
  Abs/1 -> Divide/1

== system cpp_m1hp_demo/Mount_Drv_FDR2023_linear/DRV Friction/EL DT Lugre Fr model/g(v) ==
  v : Inport
  Enable : EnablePort
  Constant : Constant  Value=0
  Sum : Sum  Inputs=|++
  gc : Constant  Value=Tc/sigma0
  gs : Subsystem
  g : Outport
  wires:
  Constant/1 -> gs/Enable
  gc/1 -> Sum/2
  gs/1(gs(v)) -> Sum/1
  v/1 -> gs/1(v)
  Sum/1 -> g/1

== system cpp_m1hp_demo/Mount_Drv_FDR2023_linear/DRV Friction/EL DT Lugre Fr model/v2z ==
  v : Inport
  g(v) : Inport  Port=2
  z : Inport  Port=3
  Enable : EnablePort
  Abs : Abs  SaturateOnIntegerOverflow=off
  Divide : Product  Inputs=*/*
  Sum : Sum  Inputs=|+-
  dz : Outport
  wires:
  z/1 -> Divide/3
  g(v)/1 -> Divide/2
  Sum/1 -> dz/1
  v/1 -> Abs/1, Sum/1
  Divide/1 -> Sum/2
  Abs/1 -> Divide/1

== system cpp_m1hp_demo/Mount_Drv_FDR2023_linear/DRV Friction/EL DT Lugre Fr model_/g(v) ==
  v : Inport
  Enable : EnablePort
  Constant : Constant  Value=0
  Sum : Sum  Inputs=|++
  gc : Constant  Value=frParStruct.Tc/frParStruct.sigm0
  gs : Subsystem
  g : Outport  VectorParamsAs1DForOutWhenUnconnected=off
  wires:
  Constant/1 -> gs/Enable
  gc/1 -> Sum/2
  gs/1(gs(v)) -> Sum/1
  v/1 -> gs/1(v)
  Sum/1 -> g/1

== system cpp_m1hp_demo/Mount_Drv_FDR2023_linear/DRV Friction/EL DT Lugre Fr model_/v2z ==
  v : Inport
  g(v) : Inport  Port=2
  z : Inport  Port=3
  Enable : EnablePort
  Abs : Abs  SaturateOnIntegerOverflow=off
  Divide : Product  Inputs=*/*
  Sum : Sum  Inputs=|+-
  dz : Outport  VectorParamsAs1DForOutWhenUnconnected=off
  wires:
  z/1 -> Divide/3
  g(v)/1 -> Divide/2
  Sum/1 -> dz/1
  v/1 -> Abs/1, Sum/1
  Divide/1 -> Sum/2
  Abs/1 -> Divide/1

== system cpp_m1hp_demo/Mount_Drv_FDR2023_linear/DRV Friction/GIR DT Lugre Fr model/g(v) ==
  v : Inport
  Constant : Constant  Value=0
  Sum : Sum  Inputs=|++
  gc : Constant  Value=Tc/sigma0
  gs : Subsystem
  g : Outport
  wires:
  Constant/1 -> gs/Enable
  gc/1 -> Sum/2
  gs/1(gs(v)) -> Sum/1
  v/1 -> gs/1(v)
  Sum/1 -> g/1

== system cpp_m1hp_demo/Mount_Drv_FDR2023_linear/DRV Friction/GIR DT Lugre Fr model/v2z ==
  v : Inport
  g(v) : Inport  Port=2
  z : Inport  Port=3
  Abs : Abs  SaturateOnIntegerOverflow=off
  Divide : Product  Inputs=*/*
  Sum : Sum  Inputs=|+-
  dz : Outport
  wires:
  z/1 -> Divide/3
  g(v)/1 -> Divide/2
  Sum/1 -> dz/1
  v/1 -> Abs/1, Sum/1
  Divide/1 -> Sum/2
  Abs/1 -> Divide/1

== system cpp_m1hp_demo/Mount_Drv_FDR2023_linear/DRV Friction/GIR DT Lugre Fr model_/g(v) ==
  v : Inport
  Constant : Constant  Value=0
  Sum : Sum  Inputs=|++
  gc : Constant  Value=frParStruct.Tc/frParStruct.sigm0
  gs : Subsystem
  g : Outport  VectorParamsAs1DForOutWhenUnconnected=off
  wires:
  Constant/1 -> gs/Enable
  gc/1 -> Sum/2
  gs/1(gs(v)) -> Sum/1
  v/1 -> gs/1(v)
  Sum/1 -> g/1

== system cpp_m1hp_demo/Mount_Drv_FDR2023_linear/DRV Friction/GIR DT Lugre Fr model_/v2z ==
  note: $\text{Let}\\ |v| = v \sign(v) \\ \text{Sign function approximation:}\\ S_0(v) = \frac{2}{\pi}\atan(k_v v) \\ \text{Then, one approximates the original LuGre model equation}\\ \dot{z} = v - \frac{|v|}{g(v)}z \\ \text{with} \\ \dot{z} = vS_0^2(v) - \frac{vS_0(v)}{g(v)}z .$
  note: Original implementation
  v : Inport
  g(v) : Inport  Port=2
  z : Inport  Port=3
  2/pi : Gain  Gain=2/pi
  Abs1 : Abs  SaturateOnIntegerOverflow=off
  Divide : Product  Inputs=*/*
  Divide1 : Product  Inputs=*/*
  Divide2 : Product  Inputs=**
  Divide3 : Product  Inputs=**
  Math Function : Math  Operator=square  SignedPower=on
  Smoothed-Discontinuous Lugre Model Switch : ManualSwitch
  Sum : Sum  Inputs=|+-
  Sum1 : Sum  Inputs=|+-
  Trigonometric Function : Trigonometry  Operator=atan
  kv : Gain  Gain=1e6%1e-6
  dz : Outport  VectorParamsAs1DForOutWhenUnconnected=off
  wires:
  Smoothed-Discontinuous Lugre Model Switch/1 -> dz/1
  Sum/1 -> Smoothed-Discontinuous Lugre Model Switch/1  "Smoothed Lugre"
  Divide2/1 -> Sum/1
  Divide3/1 -> Divide/1  "S_2"
  Math Function/1 -> Divide2/2  "S_1"
  2/pi/1 -> Math Function/1, Divide3/1  "S_0"
  kv/1 -> Trigonometric Function/1
  Trigonometric Function/1 -> 2/pi/1
  v/1 -> Divide2/1, kv/1, Divide3/2, Sum1/1, Abs1/1
  z/1 -> Divide/3, Divide1/3
  Sum1/1 -> Smoothed-Discontinuous Lugre Model Switch/2  "Discontinuous"
  Abs1/1 -> Divide1/1
  g(v)/1 -> Divide/2, Divide1/2
  Divide1/1 -> Sum1/2
  Divide/1 -> Sum/2

== system cpp_m1hp_demo/Mount_Drv_FDR2023_linear/Friction/Friction Alt/g(v) ==
  v : Inport
  Enable : EnablePort
  Constant : Constant  Value=0
  Sum : Sum  Inputs=|++
  gc : Constant  Value=Tc/sigma0
  gs : Subsystem
  g : Outport
  wires:
  Sum/1 -> g/1
  v/1 -> gs/1(v)
  gs/1(gs(v)) -> Sum/1
  gc/1 -> Sum/2
  Constant/1 -> gs/Enable

== system cpp_m1hp_demo/Mount_Drv_FDR2023_linear/Friction/Friction Alt/v2z ==
  v : Inport
  g(v) : Inport  Port=2
  z : Inport  Port=3
  Enable : EnablePort
  Abs : Abs  SaturateOnIntegerOverflow=off
  Divide : Product  Inputs=*/*
  Sum : Sum  Inputs=|+-
  dz : Outport
  wires:
  Abs/1 -> Divide/1
  Divide/1 -> Sum/2
  v/1 -> Sum/1, Abs/1
  Sum/1 -> dz/1
  g(v)/1 -> Divide/2
  z/1 -> Divide/3

== system cpp_m1hp_demo/Mount_Drv_FDR2023_linear/Friction/Friction Az/g(v) ==
  v : Inport
  Enable : EnablePort
  Constant : Constant  Value=0
  Sum : Sum  Inputs=|++
  gc : Constant  Value=Tc/sigma0
  gs : Subsystem
  g : Outport
  wires:
  Sum/1 -> g/1
  v/1 -> gs/1(v)
  gs/1(gs(v)) -> Sum/1
  gc/1 -> Sum/2
  Constant/1 -> gs/Enable

== system cpp_m1hp_demo/Mount_Drv_FDR2023_linear/Friction/Friction Az/v2z ==
  v : Inport
  g(v) : Inport  Port=2
  z : Inport  Port=3
  Enable : EnablePort
  Abs : Abs  SaturateOnIntegerOverflow=off
  Divide : Product  Inputs=*/*
  Sum : Sum  Inputs=|+-
  dz : Outport
  wires:
  Abs/1 -> Divide/1
  Divide/1 -> Sum/2
  v/1 -> Sum/1, Abs/1
  Sum/1 -> dz/1
  g(v)/1 -> Divide/2
  z/1 -> Divide/3

== system cpp_m1hp_demo/Mount_Drv_FDR2023_linear/Friction/Friction Gir/PT1 ==
  in : Inport
  Transfer Fcn : TransferFcn  Denominator=[1/(2*pi*f) 1]
  out : Outport
  wires:
  in/1 -> Transfer Fcn/1
  Transfer Fcn/1 -> out/1

== system cpp_m1hp_demo/Mount_Drv_FDR2023_linear/Friction/Friction Gir/g(v) ==
  v : Inport
  Constant : Constant  Value=0
  Sum : Sum  Inputs=|++
  gc : Constant  Value=Tc/sigma0
  gs : Subsystem
  g : Outport
  wires:
  Sum/1 -> g/1
  v/1 -> gs/1(v)
  gs/1(gs(v)) -> Sum/1
  gc/1 -> Sum/2
  Constant/1 -> gs/Enable

== system cpp_m1hp_demo/Mount_Drv_FDR2023_linear/Friction/Friction Gir/v2z ==
  v : Inport
  g(v) : Inport  Port=2
  z : Inport  Port=3
  Abs : Abs  SaturateOnIntegerOverflow=off
  Divide : Product  Inputs=*/*
  Sum : Sum  Inputs=|+-
  dz : Outport
  wires:
  Abs/1 -> Divide/1
  Divide/1 -> Sum/2
  v/1 -> Sum/1, Abs/1
  Sum/1 -> dz/1
  g(v)/1 -> Divide/2
  z/1 -> Divide/3

== system cpp_m1hp_demo/Mount_Drv_FDR2023_linear/Parasitic torque model/Parasitic AZ/For Each Subsystem ==
  In1 : Inport  Partition=on  PartitionDimension=1  PartitionWidth=1  PartitionOffset=0
  EMF Spatial Pattern (N/A) : Sin  TimeSource=Use external signal  Amplitude=oParasitic.oEmf.SpAmp_NPerA  Frequency=oParasitic.oEmf.SpFreq_mmInv*2*pi  Phase=oParasitic.oEmf.SpPhase_rad  SampleTime=0
  For Each : ForEach  DisableCoverage=on
  Sum of Elements2 : Sum  Inputs=+
  Out1 : Outport  ConcatenationDimension=1
  wires:
  Sum of Elements2/1 -> Out1/1
  In1/1 -> EMF Spatial Pattern (N/A)/1
  EMF Spatial Pattern (N/A)/1 -> Sum of Elements2/1

== system cpp_m1hp_demo/Mount_Drv_FDR2023_linear/Parasitic torque model/Parasitic AZ/For Each Subsystem1 ==
  In1 : Inport  Partition=on  PartitionDimension=1  PartitionWidth=1  PartitionOffset=0
  Cogging Spatial Pattern (N) : Sin  TimeSource=Use external signal  Amplitude=oParasitic.oCog.SpAmp_N  Frequency=oParasitic.oCog.SpFreq_mmInv*2*pi  Phase=oParasitic.oCog.SpPhase_rad  SampleTime=0
  For Each : ForEach  DisableCoverage=on
  Sum of Elements2 : Sum  Inputs=+
  Out1 : Outport  ConcatenationDimension=1
  wires:
  Sum of Elements2/1 -> Out1/1
  In1/1 -> Cogging Spatial Pattern (N)/1
  Cogging Spatial Pattern (N)/1 -> Sum of Elements2/1

== system cpp_m1hp_demo/Mount_Drv_FDR2023_linear/Parasitic torque model/Parasitic EL/For Each Subsystem ==
  In1 : Inport  Partition=on  PartitionDimension=1  PartitionWidth=1  PartitionOffset=0
  EMF Spatial Pattern (N/A) : Sin  TimeSource=Use external signal  Amplitude=oParasitic.oEmf.SpAmp_NPerA  Frequency=oParasitic.oEmf.SpFreq_mmInv*2*pi  Phase=oParasitic.oEmf.SpPhase_rad  SampleTime=0
  For Each : ForEach  DisableCoverage=on
  Sum of Elements2 : Sum  Inputs=+
  Out1 : Outport  ConcatenationDimension=1
  wires:
  Sum of Elements2/1 -> Out1/1
  In1/1 -> EMF Spatial Pattern (N/A)/1
  EMF Spatial Pattern (N/A)/1 -> Sum of Elements2/1

== system cpp_m1hp_demo/Mount_Drv_FDR2023_linear/Parasitic torque model/Parasitic EL/For Each Subsystem1 ==
  In1 : Inport  Partition=on  PartitionDimension=1  PartitionWidth=1  PartitionOffset=0
  Cogging Spatial Pattern (N) : Sin  TimeSource=Use external signal  Amplitude=oParasitic.oCog.SpAmp_N  Frequency=oParasitic.oCog.SpFreq_mmInv*2*pi  Phase=oParasitic.oCog.SpPhase_rad  SampleTime=0
  For Each : ForEach  DisableCoverage=on
  Sum of Elements2 : Sum  Inputs=+
  Out1 : Outport  ConcatenationDimension=1
  wires:
  Sum of Elements2/1 -> Out1/1
  In1/1 -> Cogging Spatial Pattern (N)/1
  Cogging Spatial Pattern (N)/1 -> Sum of Elements2/1

== system cpp_m1hp_demo/Mount_Drv_FDR2023_linear/Parasitic torque model/Parasitic GIR/For Each Subsystem ==
  In1 : Inport  Partition=on  PartitionDimension=1  PartitionWidth=1  PartitionOffset=0
  (N/A) : Sin  TimeSource=Use external signal  Amplitude=oParasitic.oEmf.SpAmp_NmPerA  Frequency=oParasitic.oEmf.SpFreq_degInv*2*pi  Phase=oParasitic.oEmf.SpPhase_rad  SampleTime=0
  For Each : ForEach  DisableCoverage=on
  Sum of Elements2 : Sum  Inputs=+
  Out1 : Outport  ConcatenationDimension=1
  wires:
  Sum of Elements2/1 -> Out1/1
  In1/1 -> (N/A)/1
  (N/A)/1 -> Sum of Elements2/1

== system cpp_m1hp_demo/Mount_Drv_FDR2023_linear/Parasitic torque model/Parasitic GIR/For Each Subsystem1 ==
  In1 : Inport  Partition=on  PartitionDimension=1  PartitionWidth=1  PartitionOffset=0
  Cogging Spatial Pattern (N) : Sin  TimeSource=Use external signal  Amplitude=oParasitic.oCog.SpAmp_Nm  Frequency=oParasitic.oCog.SpFreq_degInv*2*pi  Phase=oParasitic.oCog.SpPhase_rad  SampleTime=0
  For Each : ForEach  DisableCoverage=on
  Sum of Elements2 : Sum  Inputs=+
  Out1 : Outport  ConcatenationDimension=1
  wires:
  Sum of Elements2/1 -> Out1/1
  In1/1 -> Cogging Spatial Pattern (N)/1
  Cogging Spatial Pattern (N)/1 -> Sum of Elements2/1

== system cpp_m1hp_demo/Mount_Drv_FDR2023_linear/DRV Friction/AZ DT Lugre Fr mode/g(v)/gs ==
  v : Inport
  Enable : EnablePort
  Divide : Product  Inputs=**
  Gain : Gain  Gain=1/vs
  Math Function : Math  SignedPower=on
  Math Function1 : Math  Operator=magnitude^2  SignedPower=on
  Unary Minus : UnaryMinus
  gs : Constant  Value=(Ts-Tc)/sigma0
  gs(v) : Outport
  wires:
  Divide/1 -> gs(v)/1
  v/1 -> Gain/1
  Gain/1 -> Math Function1/1
  Unary Minus/1 -> Math Function/1
  Math Function1/1 -> Unary Minus/1
  gs/1 -> Divide/2
  Math Function/1 -> Divide/1

== system cpp_m1hp_demo/Mount_Drv_FDR2023_linear/DRV Friction/EL DT Lugre Fr model/g(v)/gs ==
  v : Inport
  Enable : EnablePort
  Divide : Product  Inputs=**
  Gain : Gain  Gain=1/vs
  Math Function : Math  SignedPower=on
  Math Function1 : Math  Operator=magnitude^2  SignedPower=on
  Unary Minus : UnaryMinus
  gs : Constant  Value=(Ts-Tc)/sigma0
  gs(v) : Outport
  wires:
  Divide/1 -> gs(v)/1
  v/1 -> Gain/1
  Gain/1 -> Math Function1/1
  Unary Minus/1 -> Math Function/1
  Math Function1/1 -> Unary Minus/1
  gs/1 -> Divide/2
  Math Function/1 -> Divide/1

== system cpp_m1hp_demo/Mount_Drv_FDR2023_linear/DRV Friction/EL DT Lugre Fr model_/g(v)/gs ==
  v : Inport
  Enable : EnablePort
  Divide : Product  Inputs=**
  Gain : Gain  Gain=1/frParStruct.vs
  Math Function : Math  SignedPower=on
  Math Function1 : Math  Operator=magnitude^2  SignedPower=on
  Unary Minus : UnaryMinus
  gs : Constant  Value=(frParStruct.Ts-frParStruct.Tc)/frParStruct.sigm0
  gs(v) : Outport  VectorParamsAs1DForOutWhenUnconnected=off
  wires:
  Divide/1 -> gs(v)/1
  v/1 -> Gain/1
  Gain/1 -> Math Function1/1
  Unary Minus/1 -> Math Function/1
  Math Function1/1 -> Unary Minus/1
  gs/1 -> Divide/2
  Math Function/1 -> Divide/1

== system cpp_m1hp_demo/Mount_Drv_FDR2023_linear/DRV Friction/GIR DT Lugre Fr model/g(v)/gs ==
  v : Inport
  Enable : EnablePort
  Divide : Product  Inputs=**
  Gain : Gain  Gain=1/vs
  Math Function : Math  SignedPower=on
  Math Function1 : Math  Operator=magnitude^2  SignedPower=on
  Unary Minus : UnaryMinus
  gs : Constant  Value=(Ts-Tc)/sigma0
  gs(v) : Outport
  wires:
  Divide/1 -> gs(v)/1
  v/1 -> Gain/1
  Gain/1 -> Math Function1/1
  Unary Minus/1 -> Math Function/1
  Math Function1/1 -> Unary Minus/1
  gs/1 -> Divide/2
  Math Function/1 -> Divide/1

== system cpp_m1hp_demo/Mount_Drv_FDR2023_linear/DRV Friction/GIR DT Lugre Fr model_/g(v)/gs ==
  v : Inport
  Enable : EnablePort
  Divide : Product  Inputs=**
  Gain : Gain  Gain=1/frParStruct.vs
  Math Function : Math  SignedPower=on
  Math Function1 : Math  Operator=magnitude^2  SignedPower=on
  Unary Minus : UnaryMinus
  gs : Constant  Value=(frParStruct.Ts-frParStruct.Tc)/frParStruct.sigm0
  gs(v) : Outport  VectorParamsAs1DForOutWhenUnconnected=off
  wires:
  Divide/1 -> gs(v)/1
  v/1 -> Gain/1
  Gain/1 -> Math Function1/1
  Unary Minus/1 -> Math Function/1
  Math Function1/1 -> Unary Minus/1
  gs/1 -> Divide/2
  Math Function/1 -> Divide/1

== system cpp_m1hp_demo/Mount_Drv_FDR2023_linear/Friction/Friction Alt/g(v)/gs ==
  v : Inport
  Enable : EnablePort
  Divide : Product  Inputs=**
  Gain : Gain  Gain=1/vs
  Math Function : Math  SignedPower=on
  Math Function1 : Math  Operator=magnitude^2  SignedPower=on
  Unary Minus : UnaryMinus
  gs : Constant  Value=(Ts-Tc)/sigma0
  gs(v) : Outport
  wires:
  Math Function/1 -> Divide/1
  gs/1 -> Divide/2
  Math Function1/1 -> Unary Minus/1
  Unary Minus/1 -> Math Function/1
  Gain/1 -> Math Function1/1
  v/1 -> Gain/1
  Divide/1 -> gs(v)/1

== system cpp_m1hp_demo/Mount_Drv_FDR2023_linear/Friction/Friction Az/g(v)/gs ==
  v : Inport
  Enable : EnablePort
  Divide : Product  Inputs=**
  Gain : Gain  Gain=1/vs
  Math Function : Math  SignedPower=on
  Math Function1 : Math  Operator=magnitude^2  SignedPower=on
  Unary Minus : UnaryMinus
  gs : Constant  Value=(Ts-Tc)/sigma0
  gs(v) : Outport
  wires:
  Math Function/1 -> Divide/1
  gs/1 -> Divide/2
  Math Function1/1 -> Unary Minus/1
  Unary Minus/1 -> Math Function/1
  Gain/1 -> Math Function1/1
  v/1 -> Gain/1
  Divide/1 -> gs(v)/1
